simulink model "Lab6_Ris_2_25"  (Simulink 10.2)
settings: Solver=VariableStepAuto  StartTime=0.0  StopTime=inf  RelTol=1e-3
undefined symbols (not defined in the file): doppler, pskmod
libraries: commdigbbndpm3 x2, commeq3 x1, commsink2 x1, commrandsrc3 x1, commchan3 x1
settings Model: Creator=Newtr  LastModifiedBy=Newtr
settings DataIOCC: SaveFormat=Dataset  SignalLoggingSaveFormat=Dataset  ReturnWorkspaceOutputs=on
settings OptimizationCC: LifeSpan=auto
settings DebuggingCC: UnderspecifiedInitializationDetection=Simplified  MergeDetectMultiDrivingBlocksExec=error  FcnCallInpInsideContextMsg=error  SFUnexpectedBacktrackingDiag=error  SFNoUnconditionalDefaultTransitionDiag=error  SFExecutionAtInitializationDiag=warning  ArithmeticOperatorsInVariantConditions=error
settings HardwareCC: ProdBitPerPointer=64  ProdBitPerSizeT=64  ProdBitPerPtrDiffT=64  ProdLargestAtomicFloat=Float  ProdIntDivRoundTo=Zero  ProdEndianess=LittleEndian  ProdWordSize=64  ProdHWDeviceType=Intel->x86-64 (Windows64)
settings ModelReferenceCC: PropagateSignalLabelsOutOfModel=on
settings SFSimCC: SimUseLocalCustomCode=on  CustomCodeUndefinedFunction=FilterOut
settings RTWCC: RTWUseLocalCustomCode=on
settings CodeAppCC: StateflowObjectComments=off
settings GRTTargetCC: TargetLangStandard=C99 (ISO)  CombineOutputUpdateFcns=on  GRTInterface=off
settings ConfigComp: CovMetricSettings=dwe  CovSaveCumulativeToWorkspaceVar=off  CovSaveSingleToWorkspaceVar=off  CovExternalEMLEnable=on

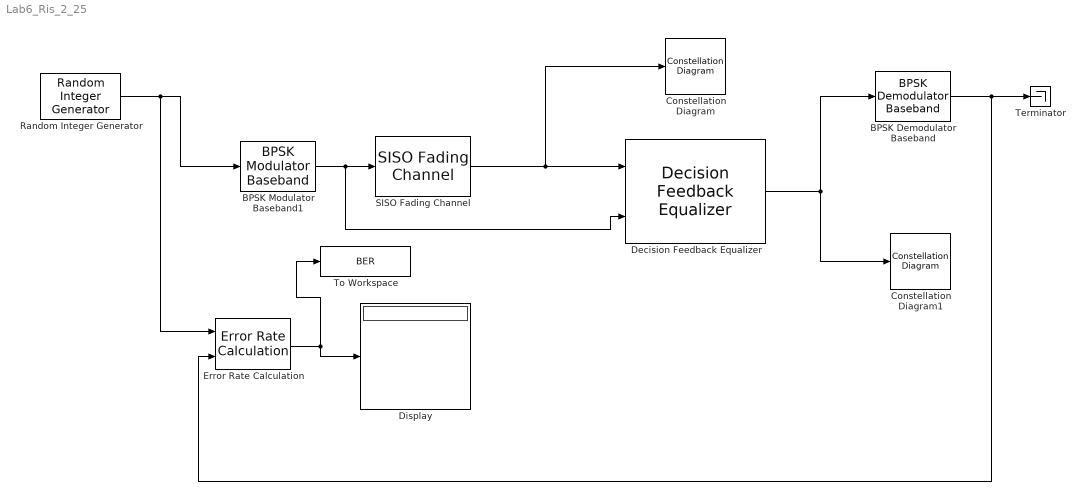
== system Lab6_Ris_2_25 ==
  BPSK Demodulator Baseband : commdigbbndpm3/BPSK Demodulator Baseband  DecType=Hard decision  VarSource=Dialog  Variance=1  Ph=0  outDtype=Inherit via internal rule  derotateFactorWordLen=16  derotateFactorDataTypeStr=Inherit: Same word length as input  derotateFactorLastDataTypeStr=Inherit: Same word length as input
  BPSK Modulator Baseband1 : commdigbbndpm3/BPSK Modulator Baseband  Ph=0  outDtype=double  outWordLen=16  outUDDataType=sfix(16)  outFracLenMode=Best precision  outFracLen=15  outDataTypeStr=double  outLastDataTypeStr=double
  Constellation Diagram : ConstellationDiagram
  Constellation Diagram1 : ConstellationDiagram
  Decision Feedback Equalizer : commeq3/Decision Feedback Equalizer  NumForwardTaps=4  NumFeedbackTaps=4  Constellation=pskmod( [0:1],2 )  InputSamplesPerSymbol=1  Algorithm=LMS  StepSize=0.1  ForgettingFactor=0.99  InitialInverseCorrelationMatrix=0.1  ReferenceTap=2  InputDelay=0  AdaptWeightsSource=Property  AdaptWeights=on  InitialWeightsSource=Auto  InitialWeights=0  TrainingInitialWeights=0  BlindInitialWeights=[ 0; 0; 1; 0; 0; 0; 0; 0 ]  WeightUpdatePeriod=1  TrainingFlagInputPort=off  AdaptAfterTraining=on  ResetInputPort=off  ErrorOutputPort=off  TapWeightsOutputPort=off  SimulateUsing=Code generation
      settings: SourceProductBaseCode=CM
  Display : Display
  Error Rate Calculation : commsink2/Error Rate Calculation  N=0  st_delay=0  cp_mode=Entire frame  subframe=[]  PMode=Port  WsName=ErrorVec  RsMode2=off  stop=on  numErr=200  maxBits=500
  Random Integer Generator : commrandsrc3/Random Integer Generator  SetSize=2  SeedSource=Auto  Seed=0  SampleTime=1/500000  SamplesPerFrame=8  OutputDataType=double  SimulateUsing=Interpreted execution
  SISO Fading Channel : commchan3/SISO Fading Channel  InheritSampleRate=on  SampleRate=1  PathDelays=1.0e-004*[0 0.0400 0.0800 0.1200]  AveragePathGains=[0 -3 -6 -9]  NormalizePathGains=on  FadingDistribution=Rician  KFactor=10  DirectPathDopplerShift=0  DirectPathInitialPhase=0  MaximumDopplerShift=200  DopplerSpectrum=doppler('Jakes')  RandomStream=mt19937ar with seed  Seed=73  PathGainsOutputPort=off  ChannelFilterDelayOutputPort=off  SimulateUsing=Interpreted execution  Visualization=Off  PathsForDopplerDisplay=1  SamplesToDisplay=25%
  Terminator : Terminator
  To Workspace : ToWorkspace  VariableName=BER  SaveFormat=Timeseries  SampleTime=-1
  wires:
  Random Integer Generator/1 -> Error Rate Calculation/1, BPSK Modulator Baseband1/1
  BPSK Modulator Baseband1/1 -> SISO Fading Channel/1, Decision Feedback Equalizer/2
  Error Rate Calculation/1 -> To Workspace/1, Display/1
  SISO Fading Channel/1 -> Constellation Diagram/1, Decision Feedback Equalizer/1
  Decision Feedback Equalizer/1 -> BPSK Demodulator Baseband/1, Constellation Diagram1/1
  BPSK Demodulator Baseband/1 -> Error Rate Calculation/2, Terminator/1
